simulink model "Copy_of_Mars_capture_sim"  (R2024b)
settings: Solver=VariableStepAuto  StartTime=0.0  StopTime=5e5  MaxStep=50  RelTol=1e-6
values from neighbouring files (symbols this model uses):
  mars_escape_data = escape(Mars_planet,orbit_data,transfer_inbound_data,escape_burn_time)    [Mars_escape_setup.m]
settings Model: Creator=cpero  LastModifiedBy=cpero

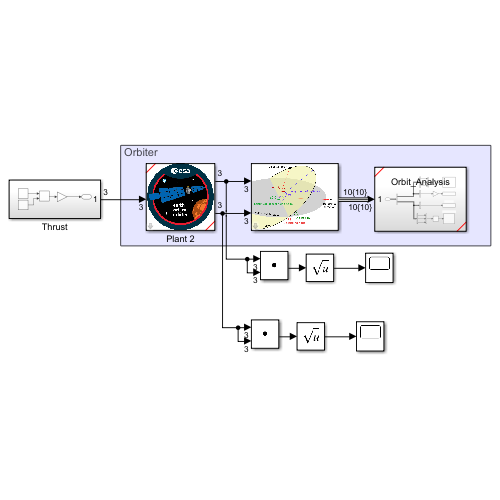
[thumbnail: Simulink's stored preview of the top-level diagram]
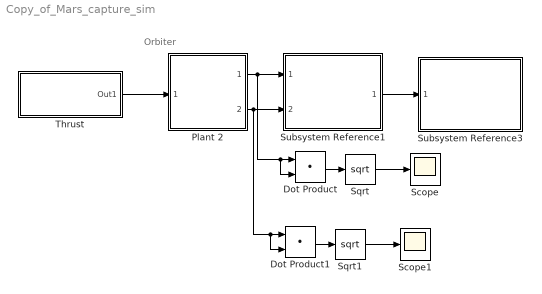
== system Copy_of_Mars_capture_sim ==
  note: Orbiter
  Dot Product : DotProduct  OutDataTypeStr=Inherit: Inherit via internal rule
  Dot Product1 : DotProduct  OutDataTypeStr=Inherit: Inherit via internal rule
  Plant 2 : Subsystem  ReferencedSubsystem=Plant  setup=mars_escape_data.initial  switch_time=0  mu=Mars_planet.mu
  Scope : Scope
  Scope1 : Scope
  Sqrt : Sqrt
  Sqrt1 : Sqrt
  Subsystem Reference1 : Subsystem  ReferencedSubsystem=Orbit_Calculations  mu=Mars_planet.mu
  Subsystem Reference3 : Subsystem  ReferencedSubsystem=Orbit_Analysis
  Thrust : Subsystem
  wires:
  Plant 2/1 -> Dot Product/2, Dot Product/1, Subsystem Reference1/1
  Subsystem Reference1/1 -> Subsystem Reference3/1
  Dot Product/1 -> Sqrt/1
  Sqrt/1 -> Scope/1
  Thrust/1(Out1) -> Plant 2/1
  Dot Product1/1 -> Sqrt1/1
  Plant 2/2 -> Dot Product1/2, Dot Product1/1, Subsystem Reference1/2
  Sqrt1/1 -> Scope1/1

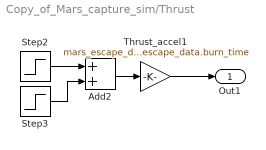
== system Copy_of_Mars_capture_sim/Thrust ==
  Add2 : Sum
  Step2 : Step  Time=mars_escape_data.time  SampleTime=0
  Step3 : Step  Time=mars_escape_data.time + mars_escape_data.burn_time  After=-1  SampleTime=0
  Thrust_accel1 : Gain  Gain=mars_escape_data.v_target/mars_escape_data.burn_time
  Out1 : Outport
  wires:
  Step3/1 -> Add2/2
  Add2/1 -> Thrust_accel1/1
  Thrust_accel1/1 -> Out1/1
  Step2/1 -> Add2/1
